simulink model "subsistema_hoist"  (R2023b)
settings: Solver=VariableStepAuto  StartTime=0.0  StopTime=10.0  RelTol=1e-3
undefined symbols (not defined in the file): bcx, bcy, bhb, bhd, bhEb, bhm, bhwu, g, Hc, ih, J_hd_hEb, J_hm_hb, Kcy, khwu, Lh0, Ms, rhd, Thb_Max, ThEb_Max, Yt0
settings Model: Creator=Nahuel  LastModifiedBy=rodri

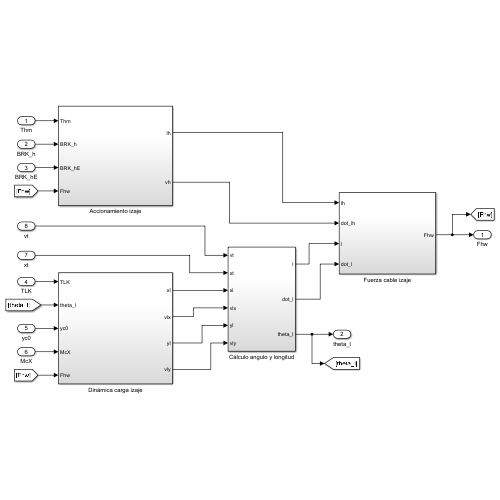
[thumbnail: Simulink's stored preview of the top-level diagram]
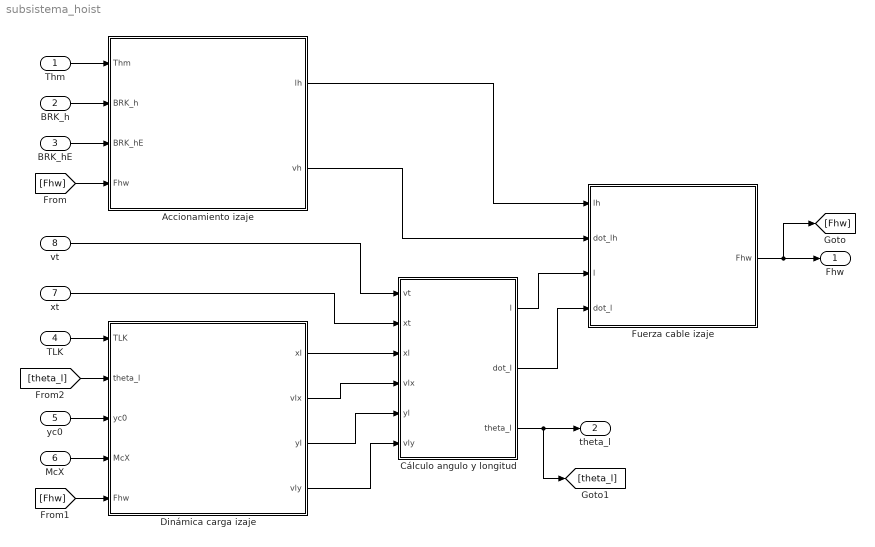
== system subsistema_hoist ==
  Thm : Inport
  BRK_h : Inport  Port=2
  BRK_hE : Inport  Port=3
  TLK : Inport  Port=4
  yc0 : Inport  Port=5
  McX : Inport  Port=6
  xt : Inport  Port=7
  vt : Inport  Port=8
  Accionamiento izaje : Subsystem
  Cálculo angulo y longitud : Subsystem
  Dinámica carga izaje : Subsystem
  Fuerza cable izaje : Subsystem
  Fhw : Outport
  theta_l : Outport  Port=2
  wires:
  Thm/1 -> Accionamiento izaje/1(Thm)
  BRK_h/1 -> Accionamiento izaje/2(BRK_h)
  BRK_hE/1 -> Accionamiento izaje/3(BRK_hE)
  Accionamiento izaje/1(lh) -> Fuerza cable izaje/1(lh)
  Accionamiento izaje/2(vh) -> Fuerza cable izaje/2(dot_lh)
  Fuerza cable izaje/1(Fhw) -> Fhw/1, [Fhw]
  [Fhw] -> Accionamiento izaje/4(Fhw)
  TLK/1 -> Dinámica carga izaje/1(TLK)
  yc0/1 -> Dinámica carga izaje/3(yc0)
  McX/1 -> Dinámica carga izaje/4(McX)
  [Fhw] -> Dinámica carga izaje/5(Fhw)
  Dinámica carga izaje/1(xl) -> Cálculo angulo y longitud/3(xl)
  xt/1 -> Cálculo angulo y longitud/2(xt)
  Dinámica carga izaje/2(vlx) -> Cálculo angulo y longitud/4(vlx)
  Dinámica carga izaje/3(yl) -> Cálculo angulo y longitud/5(yl)
  Dinámica carga izaje/4(vly) -> Cálculo angulo y longitud/6(vly)
  vt/1 -> Cálculo angulo y longitud/1(vt)
  Cálculo angulo y longitud/1(l) -> Fuerza cable izaje/3(l)
  Cálculo angulo y longitud/2(dot_l) -> Fuerza cable izaje/4(dot_l)
  Cálculo angulo y longitud/3(theta_l) -> theta_l/1, [theta_l]
  [theta_l] -> Dinámica carga izaje/2(theta_l)

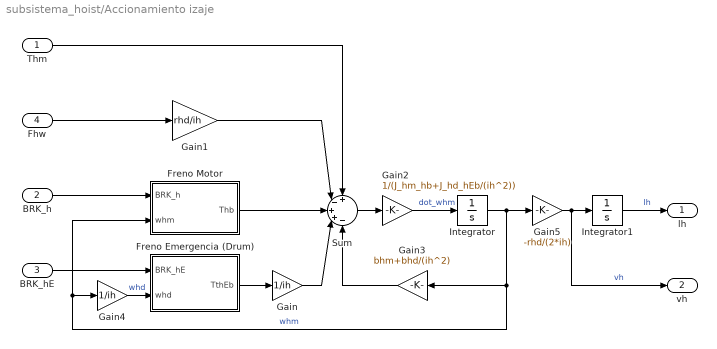
== system subsistema_hoist/Accionamiento izaje ==
  Thm : Inport
  BRK_h : Inport  Port=2
  BRK_hE : Inport  Port=3
  Fhw : Inport  Port=4
  Freno Emergencia (Drum) : Subsystem
  Freno Motor : Subsystem
  Gain : Gain  Gain=1/ih
  Gain1 : Gain  Gain=rhd/ih
  Gain2 : Gain  Gain=1/(J_hm_hb+J_hd_hEb/(ih^2))
  Gain3 : Gain  Gain=bhm+bhd/(ih^2)
  Gain4 : Gain  Gain=1/ih
  Gain5 : Gain  Gain=-rhd/(2*ih)
  Integrator : Integrator
  Integrator1 : Integrator
  Sum : Sum  Inputs=+-++-
  lh : Outport
  vh : Outport  Port=2
  wires:
  Gain5/1 -> Integrator1/1, vh/1  "vh"
  Integrator/1 -> Gain5/1, Gain3/1, Freno Motor/2(whm), Gain4/1  "whm"
  Freno Emergencia (Drum)/1(TthEb) -> Gain/1
  Gain3/1 -> Sum/5
  Thm/1 -> Sum/1
  BRK_h/1 -> Freno Motor/1(BRK_h)
  Gain/1 -> Sum/4
  Gain2/1 -> Integrator/1  "dot_whm"
  Sum/1 -> Gain2/1
  Gain4/1 -> Freno Emergencia (Drum)/2(whd)  "whd"
  BRK_hE/1 -> Freno Emergencia (Drum)/1(BRK_hE)
  Fhw/1 -> Gain1/1
  Freno Motor/1(Thb) -> Sum/3
  Gain1/1 -> Sum/2
  Integrator1/1 -> lh/1  "lh"

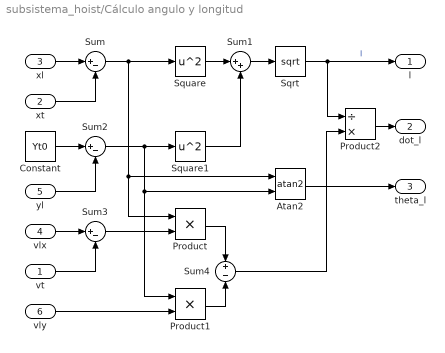
== system subsistema_hoist/Cálculo angulo y longitud ==
  vt : Inport
  xt : Inport  Port=2
  xl : Inport  Port=3
  vlx : Inport  Port=4
  yl : Inport  Port=5
  vly : Inport  Port=6
  Atan2 : Trigonometry  Operator=atan2
  Constant : Constant  Value=Yt0
  Product : Product
  Product1 : Product
  Product2 : Product  Inputs=/*
  Sqrt : Sqrt
  Square : Math  Operator=square
  Square1 : Math  Operator=square
  Sum : Sum  Inputs=|+-
  Sum1 : Sum  Inputs=|++
  Sum2 : Sum  Inputs=|+-
  Sum3 : Sum  Inputs=|+-
  Sum4 : Sum  Inputs=+-
  l : Outport
  dot_l : Outport  Port=2
  theta_l : Outport  Port=3
  wires:
  Product2/1 -> dot_l/1
  Sqrt/1 -> l/1, Product2/1  "l"
  Sum1/1 -> Sqrt/1
  Sum2/1 -> Product1/1, Atan2/2, Square1/1
  Sum/1 -> Product/1, Atan2/1, Square/1
  yl/1 -> Sum2/2
  Atan2/1 -> theta_l/1
  vly/1 -> Product1/2
  xl/1 -> Sum/1
  Constant/1 -> Sum2/1
  Sum3/1 -> Product/2
  Square1/1 -> Sum1/2
  vt/1 -> Sum3/2
  Sum4/1 -> Product2/2
  vlx/1 -> Sum3/1
  xt/1 -> Sum/2
  Square/1 -> Sum1/1
  Product1/1 -> Sum4/2
  Product/1 -> Sum4/1

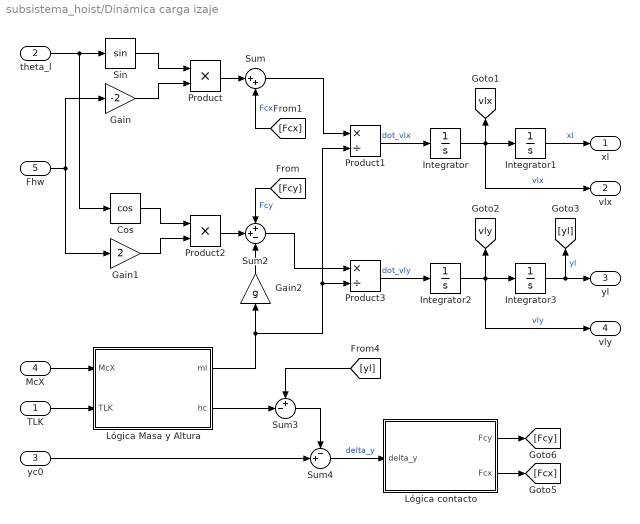
== system subsistema_hoist/Dinámica carga izaje ==
  TLK : Inport
  theta_l : Inport  Port=2
  yc0 : Inport  Port=3
  McX : Inport  Port=4
  Fhw : Inport  Port=5
  Cos : Trigonometry  Operator=cos
  Gain : Gain  Gain=-2
  Gain1 : Gain  Gain=2
  Gain2 : Gain  Gain=g
  Integrator{,1..3} (4 alike) : Integrator
  Lógica Masa y Altura : Subsystem
  Lógica contacto : Subsystem
  Product : Product
  Product1 : Product  Inputs=*/
  Product2 : Product
  Product3 : Product  Inputs=*/
  Sin : Trigonometry
  Sum : Sum  Inputs=|++
  Sum2 : Sum  Inputs=++-
  Sum3 : Sum  Inputs=+-|
  Sum4 : Sum  Inputs=-+|
  xl : Outport
  vlx : Outport  Port=2
  yl : Outport  Port=3
  vly : Outport  Port=4
  tag scope: vlx=global, vly=global
  wires:
  theta_l/1 -> Sin/1, Cos/1
  Integrator/1 -> vlx/1, Integrator1/1, [vlx]  "vlx"
  Sum3/1 -> Sum4/1
  Sin/1 -> Product/1
  Gain/1 -> Product/2
  [Fcy] -> Sum2/1  "Fcy"
  Integrator2/1 -> vly/1, Integrator3/1, [vly]  "vly"
  Integrator3/1 -> yl/1, [yl]  "yl"
  Fhw/1 -> Gain1/1, Gain/1
  [Fcx] -> Sum/2  "Fcx"
  Product/1 -> Sum/1
  Product1/1 -> Integrator/1  "dot_vlx"
  Gain2/1 -> Sum2/3
  Cos/1 -> Product2/1
  Gain1/1 -> Product2/2
  [yl] -> Sum3/1
  Product2/1 -> Sum2/2
  yc0/1 -> Sum4/2
  Sum2/1 -> Product3/1
  Product3/1 -> Integrator2/1  "dot_vly"
  Sum/1 -> Product1/1
  Integrator1/1 -> xl/1  "xl"
  Sum4/1 -> Lógica contacto/1(delta_y)  "delta_y"
  Lógica contacto/1(Fcy) -> [Fcy]
  Lógica contacto/2(Fcx) -> [Fcx]
  Lógica Masa y Altura/1(ml) -> Product1/2, Product3/2, Gain2/1
  McX/1 -> Lógica Masa y Altura/1(McX)
  TLK/1 -> Lógica Masa y Altura/2(TLK)
  Lógica Masa y Altura/2(hc) -> Sum3/2

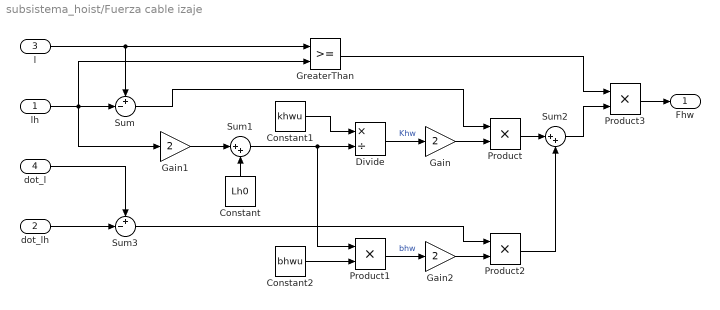
== system subsistema_hoist/Fuerza cable izaje ==
  lh : Inport
  dot_lh : Inport  Port=2
  l : Inport  Port=3
  dot_l : Inport  Port=4
  Constant : Constant  Value=Lh0
  Constant1 : Constant  Value=khwu
  Constant2 : Constant  Value=bhwu
  Divide : Product  Inputs=*/  RndMeth=Zero  SaturateOnIntegerOverflow=on
  Gain : Gain  Gain=2
  Gain1 : Gain  Gain=2
  Gain2 : Gain  Gain=2
  GreaterThan : RelationalOperator  OutDataTypeStr=boolean  RndMeth=Simplest  InputSameDT=off
  Product{,1..3} (4 alike) : Product
  Sum : Sum  Inputs=+-|
  Sum1 : Sum  Inputs=|++
  Sum2 : Sum  Inputs=|++
  Sum3 : Sum  Inputs=+-|
  Fhw : Outport
  wires:
  Constant/1 -> Sum1/2
  Constant2/1 -> Product1/2
  Sum1/1 -> Divide/2, Product1/1
  lh/1 -> Sum/2, GreaterThan/2, Gain1/1
  Product/1 -> Sum2/1
  Gain1/1 -> Sum1/1
  l/1 -> Sum/1, GreaterThan/1
  Product2/1 -> Sum2/2
  Product3/1 -> Fhw/1
  GreaterThan/1 -> Product3/1
  dot_lh/1 -> Sum3/2
  Constant1/1 -> Divide/1
  Product1/1 -> Gain2/1  "bhw"
  Sum/1 -> Product/1
  Gain2/1 -> Product2/2
  Divide/1 -> Gain/1  "Khw"
  Sum2/1 -> Product3/2
  Sum3/1 -> Product2/1
  dot_l/1 -> Sum3/1
  Gain/1 -> Product/2

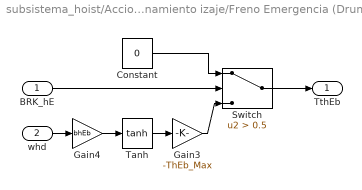
== system subsistema_hoist/Accionamiento izaje/Freno Emergencia (Drum) ==
  BRK_hE : Inport
  whd : Inport  Port=2
  Constant : Constant  Value=0
  Gain3 : Gain  Gain=-ThEb_Max
  Gain4 : Gain  Gain=bhEb
  Switch : Switch  Criteria=u2 > Threshold  Threshold=0.5  SaturateOnIntegerOverflow=off  InputSameDT=off
  Tanh : Trigonometry  Operator=tanh
  TthEb : Outport
  wires:
  BRK_hE/1 -> Switch/2
  Gain3/1 -> Switch/3
  Constant/1 -> Switch/1
  whd/1 -> Gain4/1
  Gain4/1 -> Tanh/1
  Tanh/1 -> Gain3/1
  Switch/1 -> TthEb/1

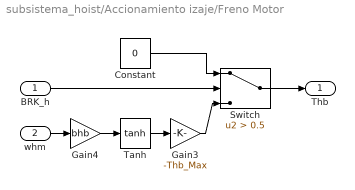
== system subsistema_hoist/Accionamiento izaje/Freno Motor ==
  BRK_h : Inport
  whm : Inport  Port=2
  Constant : Constant  Value=0
  Gain3 : Gain  Gain=-Thb_Max
  Gain4 : Gain  Gain=bhb
  Switch : Switch  Criteria=u2 > Threshold  Threshold=0.5  SaturateOnIntegerOverflow=off  InputSameDT=off
  Tanh : Trigonometry  Operator=tanh
  Thb : Outport
  wires:
  BRK_h/1 -> Switch/2
  Gain3/1 -> Switch/3
  Constant/1 -> Switch/1
  whm/1 -> Gain4/1
  Gain4/1 -> Tanh/1
  Tanh/1 -> Gain3/1
  Switch/1 -> Thb/1

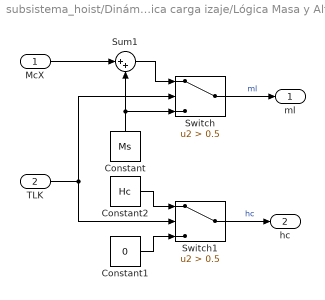
== system subsistema_hoist/Dinámica carga izaje/Lógica Masa y Altura ==
  McX : Inport
  TLK : Inport  Port=2
  Constant : Constant  Value=Ms
  Constant1 : Constant  Value=0
  Constant2 : Constant  Value=Hc
  Sum1 : Sum  Inputs=|++
  Switch : Switch  Criteria=u2 > Threshold  Threshold=0.5  SaturateOnIntegerOverflow=off  InputSameDT=off
  Switch1 : Switch  Criteria=u2 > Threshold  Threshold=0.5  SaturateOnIntegerOverflow=off  InputSameDT=off
  ml : Outport
  hc : Outport  Port=2
  wires:
  Sum1/1 -> Switch/1
  Constant2/1 -> Switch1/1
  TLK/1 -> Switch/2, Switch1/2
  Switch/1 -> ml/1  "ml"
  Constant/1 -> Switch/3, Sum1/2
  Constant1/1 -> Switch1/3
  Switch1/1 -> hc/1  "hc"
  McX/1 -> Sum1/1

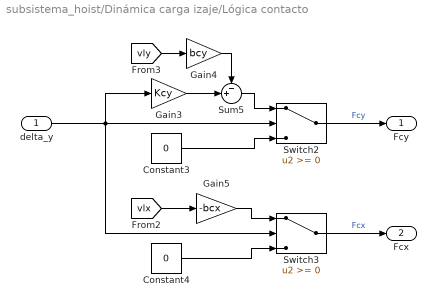
== system subsistema_hoist/Dinámica carga izaje/Lógica contacto ==
  delta_y : Inport
  Constant3 : Constant  Value=0
  Constant4 : Constant  Value=0
  Gain3 : Gain  Gain=Kcy
  Gain4 : Gain  Gain=bcy
  Gain5 : Gain  Gain=-bcx
  Sum5 : Sum  Inputs=-+|
  Switch2 : Switch  SaturateOnIntegerOverflow=off  InputSameDT=off
  Switch3 : Switch  SaturateOnIntegerOverflow=off  InputSameDT=off
  Fcy : Outport
  Fcx : Outport  Port=2
  wires:
  Sum5/1 -> Switch2/1
  [vlx] -> Gain5/1
  Gain4/1 -> Sum5/1
  [vly] -> Gain4/1
  Constant4/1 -> Switch3/3
  Gain5/1 -> Switch3/1
  Gain3/1 -> Sum5/2
  delta_y/1 -> Switch3/2, Gain3/1, Switch2/2
  Constant3/1 -> Switch2/3
  Switch2/1 -> Fcy/1  "Fcy"
  Switch3/1 -> Fcx/1  "Fcx"
